simulink model "CLSfixed_pace"  (R2024b)
settings: Solver=FixedStepAuto  StartTime=0.0  StopTime=stoptime  FixedStep=stepsize  RelTol=1e-3
undefined symbols (not defined in the file or in its folder): AVI, cfg_length, LCP_delay, LRI, pNode_length, pPath_length, PVARP, stepsize, URI, VRP
libraries: Libs_unified x157
(part 2 of 3)

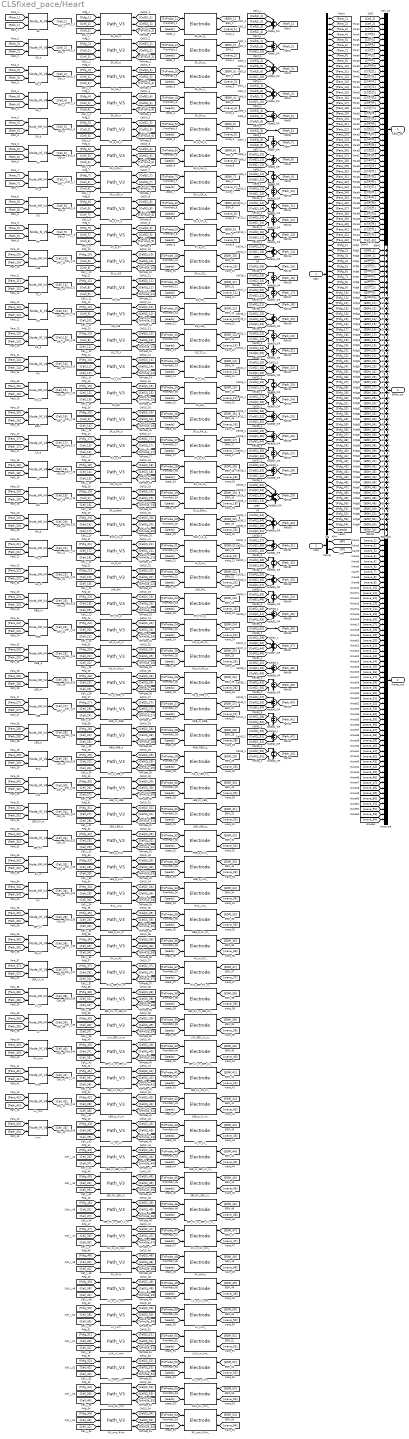
== system CLSfixed_pace/Heart ==
  Cfgin : Inport
  Pace : Inport  Port=2
  BH : Libs_unified/Node_NM_V4  SystemSampleTime=-1  VariantActivationTime=update diagram  AllowFlexibleInterface=on  Latency=0  AutoFrameSizeCalculation=off
  BH_His_p : Libs_unified/Path_V3  SystemSampleTime=-1  VariantActivationTime=update diagram  AllowFlexibleInterface=on  Latency=0  AutoFrameSizeCalculation=off
  BH_His_p_ : Libs_unified/Electrode  SystemSampleTime=-1  VariantActivationTime=update diagram  AllowFlexibleInterface=on  Latency=0  AutoFrameSizeCalculation=off
  Bach : Libs_unified/Node_M_V4  SystemSampleTime=-1  VariantActivationTime=update diagram  AllowFlexibleInterface=on  Latency=0  AutoFrameSizeCalculation=off
  Bach_LA_a : Libs_unified/Path_V3  SystemSampleTime=-1  VariantActivationTime=update diagram  AllowFlexibleInterface=on  Latency=0  AutoFrameSizeCalculation=off
  Bach_LA_a_ : Libs_unified/Electrode  SystemSampleTime=-1  VariantActivationTime=update diagram  AllowFlexibleInterface=on  Latency=0  AutoFrameSizeCalculation=off
  CN : Libs_unified/Node_N_V6  SystemSampleTime=-1  VariantActivationTime=update diagram  AllowFlexibleInterface=on  Latency=0  AutoFrameSizeCalculation=off
  CN_BH : Libs_unified/Path_V3  SystemSampleTime=-1  VariantActivationTime=update diagram  AllowFlexibleInterface=on  Latency=0  AutoFrameSizeCalculation=off
  CN_BH_ : Libs_unified/Electrode  SystemSampleTime=-1  VariantActivationTime=update diagram  AllowFlexibleInterface=on  Latency=0  AutoFrameSizeCalculation=off
  CS_LA : Libs_unified/Node_NM_V4  SystemSampleTime=-1  VariantActivationTime=update diagram  AllowFlexibleInterface=on  Latency=0  AutoFrameSizeCalculation=off
  CS_LV : Libs_unified/Node_M_V4  SystemSampleTime=-1  VariantActivationTime=update diagram  AllowFlexibleInterface=on  Latency=0  AutoFrameSizeCalculation=off
  CT : Libs_unified/Node_M_V4  SystemSampleTime=-1  VariantActivationTime=update diagram  AllowFlexibleInterface=on  Latency=0  AutoFrameSizeCalculation=off
  CT_a : Libs_unified/Node_NM_V4  SystemSampleTime=-1  VariantActivationTime=update diagram  AllowFlexibleInterface=on  Latency=0  AutoFrameSizeCalculation=off
  CT_a_CT : Libs_unified/Path_V3  SystemSampleTime=-1  VariantActivationTime=update diagram  AllowFlexibleInterface=on  Latency=0  AutoFrameSizeCalculation=off
  CT_a_CT_ : Libs_unified/Electrode  SystemSampleTime=-1  VariantActivationTime=update diagram  AllowFlexibleInterface=on  Latency=0  AutoFrameSizeCalculation=off
  Cell_out : Mux  Inputs=43
  Cfg : Demux  Outputs=[23,25,25,25,50,25,50,50,23,50,50,23,25,25,50,25,25,25,50,50,50,50,50,50,50,50,50,50,25,25,25,25,50,50,25,25,25,50,50,25,25,25,25,11,11,11,11,11,11,11,11,11,11,11,11,11,11,11,11,11,11,11,11,11,11,11,11,11,11,11,11,11,11,11,11,11,11,11,11,11,11,11,11,11,11,11,11,11,11,11,11,11,11,11,11,11,11,28]
  EGM_out : Sum  Inputs=54
  His_d : Libs_unified/Node_NM_V4  SystemSampleTime=-1  VariantActivationTime=update diagram  AllowFlexibleInterface=on  Latency=0  AutoFrameSizeCalculation=off
  His_d_LBB_m : Libs_unified/Path_V3  SystemSampleTime=-1  VariantActivationTime=update diagram  AllowFlexibleInterface=on  Latency=0  AutoFrameSizeCalculation=off
  His_d_LBB_m_ : Libs_unified/Electrode  SystemSampleTime=-1  VariantActivationTime=update diagram  AllowFlexibleInterface=on  Latency=0  AutoFrameSizeCalculation=off
  His_d_RBB_m : Libs_unified/Path_V3  SystemSampleTime=-1  VariantActivationTime=update diagram  AllowFlexibleInterface=on  Latency=0  AutoFrameSizeCalculation=off
  His_d_RBB_m_ : Libs_unified/Electrode  SystemSampleTime=-1  VariantActivationTime=update diagram  AllowFlexibleInterface=on  Latency=0  AutoFrameSizeCalculation=off
  His_m : Libs_unified/Node_NM_V4  SystemSampleTime=-1  VariantActivationTime=update diagram  AllowFlexibleInterface=on  Latency=0  AutoFrameSizeCalculation=off
  His_m_His_d : Libs_unified/Path_V3  SystemSampleTime=-1  VariantActivationTime=update diagram  AllowFlexibleInterface=on  Latency=0  AutoFrameSizeCalculation=off
  His_m_His_d_ : Libs_unified/Electrode  SystemSampleTime=-1  VariantActivationTime=update diagram  AllowFlexibleInterface=on  Latency=0  AutoFrameSizeCalculation=off
  His_p : Libs_unified/Node_NM_V4  SystemSampleTime=-1  VariantActivationTime=update diagram  AllowFlexibleInterface=on  Latency=0  AutoFrameSizeCalculation=off
  His_p_His_m : Libs_unified/Path_V3  SystemSampleTime=-1  VariantActivationTime=update diagram  AllowFlexibleInterface=on  Latency=0  AutoFrameSizeCalculation=off
  His_p_His_m_ : Libs_unified/Electrode  SystemSampleTime=-1  VariantActivationTime=update diagram  AllowFlexibleInterface=on  Latency=0  AutoFrameSizeCalculation=off
  LA : Libs_unified/Node_M_V4  SystemSampleTime=-1  VariantActivationTime=update diagram  AllowFlexibleInterface=on  Latency=0  AutoFrameSizeCalculation=off
  LA_a : Libs_unified/Node_M_V4  SystemSampleTime=-1  VariantActivationTime=update diagram  AllowFlexibleInterface=on  Latency=0  AutoFrameSizeCalculation=off
  LA_a_LA : Libs_unified/Path_V3  SystemSampleTime=-1  VariantActivationTime=update diagram  AllowFlexibleInterface=on  Latency=0  AutoFrameSizeCalculation=off
  LA_a_LA_ : Libs_unified/Electrode  SystemSampleTime=-1  VariantActivationTime=update diagram  AllowFlexibleInterface=on  Latency=0  AutoFrameSizeCalculation=off
  LBB : Libs_unified/Node_NM_V4  SystemSampleTime=-1  VariantActivationTime=update diagram  AllowFlexibleInterface=on  Latency=0  AutoFrameSizeCalculation=off
  LBB_LBB_a : Libs_unified/Path_V3  SystemSampleTime=-1  VariantActivationTime=update diagram  AllowFlexibleInterface=on  Latency=0  AutoFrameSizeCalculation=off
  LBB_LBB_a_ : Libs_unified/Electrode  SystemSampleTime=-1  VariantActivationTime=update diagram  AllowFlexibleInterface=on  Latency=0  AutoFrameSizeCalculation=off
  LBB_a : Libs_unified/Node_NM_V4  SystemSampleTime=-1  VariantActivationTime=update diagram  AllowFlexibleInterface=on  Latency=0  AutoFrameSizeCalculation=off
  LBB_a_LVA : Libs_unified/Path_V3  SystemSampleTime=-1  VariantActivationTime=update diagram  AllowFlexibleInterface=on  Latency=0  AutoFrameSizeCalculation=off
  LBB_a_LVA_ : Libs_unified/Electrode  SystemSampleTime=-1  VariantActivationTime=update diagram  AllowFlexibleInterface=on  Latency=0  AutoFrameSizeCalculation=off
  LBB_a_LV_m : Libs_unified/Path_V3  SystemSampleTime=-1  VariantActivationTime=update diagram  AllowFlexibleInterface=on  Latency=0  AutoFrameSizeCalculation=off
  LBB_a_LV_m_ : Libs_unified/Electrode  SystemSampleTime=-1  VariantActivationTime=update diagram  AllowFlexibleInterface=on  Latency=0  AutoFrameSizeCalculation=off
  LBB_m : Libs_unified/Node_NM_V4  SystemSampleTime=-1  VariantActivationTime=update diagram  AllowFlexibleInterface=on  Latency=0  AutoFrameSizeCalculation=off
  LBB_m_LBB : Libs_unified/Path_V3  SystemSampleTime=-1  VariantActivationTime=update diagram  AllowFlexibleInterface=on  Latency=0  AutoFrameSizeCalculation=off
  LBB_m_LBB_ : Libs_unified/Electrode  SystemSampleTime=-1  VariantActivationTime=update diagram  AllowFlexibleInterface=on  Latency=0  AutoFrameSizeCalculation=off
  LBB_m_SEP_LV_m : Libs_unified/Path_V3  SystemSampleTime=-1  VariantActivationTime=update diagram  AllowFlexibleInterface=on  Latency=0  AutoFrameSizeCalculation=off
  LBB_m_SEP_LV_m_ : Libs_unified/Electrode  SystemSampleTime=-1  VariantActivationTime=update diagram  AllowFlexibleInterface=on  Latency=0  AutoFrameSizeCalculation=off
  LNB : Libs_unified/Node_NM_V4  SystemSampleTime=-1  VariantActivationTime=update diagram  AllowFlexibleInterface=on  Latency=0  AutoFrameSizeCalculation=off
  LNB_BH : Libs_unified/Path_V3  SystemSampleTime=-1  VariantActivationTime=update diagram  AllowFlexibleInterface=on  Latency=0  AutoFrameSizeCalculation=off
  LNB_BH_ : Libs_unified/Electrode  SystemSampleTime=-1  VariantActivationTime=update diagram  AllowFlexibleInterface=on  Latency=0  AutoFrameSizeCalculation=off
  LV : Libs_unified/Node_NM_V4  SystemSampleTime=-1  VariantActivationTime=update diagram  AllowFlexibleInterface=on  Latency=0  AutoFrameSizeCalculation=off
  LVA : Libs_unified/Node_M_V4  SystemSampleTime=-1  VariantActivationTime=update diagram  AllowFlexibleInterface=on  Latency=0  AutoFrameSizeCalculation=off
  LVA_LV_mm : Libs_unified/Path_V3  SystemSampleTime=-1  VariantActivationTime=update diagram  AllowFlexibleInterface=on  Latency=0  AutoFrameSizeCalculation=off
  LVA_LV_mm_ : Libs_unified/Electrode  SystemSampleTime=-1  VariantActivationTime=update diagram  AllowFlexibleInterface=on  Latency=0  AutoFrameSizeCalculation=off
  LVA_SEP_LV_m : Libs_unified/Path_V3  SystemSampleTime=-1  VariantActivationTime=update diagram  AllowFlexibleInterface=on  Latency=0  AutoFrameSizeCalculation=off
  LVA_SEP_LV_m_ : Libs_unified/Electrode  SystemSampleTime=-1  VariantActivationTime=update diagram  AllowFlexibleInterface=on  Latency=0  AutoFrameSizeCalculation=off
  LV_LVm : Libs_unified/Path_V3  SystemSampleTime=-1  VariantActivationTime=update diagram  AllowFlexibleInterface=on  Latency=0  AutoFrameSizeCalculation=off
  LV_LVm_ : Libs_unified/Electrode  SystemSampleTime=-1  VariantActivationTime=update diagram  AllowFlexibleInterface=on  Latency=0  AutoFrameSizeCalculation=off
  LV_m : Libs_unified/Node_NM_V4  SystemSampleTime=-1  VariantActivationTime=update diagram  AllowFlexibleInterface=on  Latency=0  AutoFrameSizeCalculation=off
  LV_m_LV : Libs_unified/Path_V3  SystemSampleTime=-1  VariantActivationTime=update diagram  AllowFlexibleInterface=on  Latency=0  AutoFrameSizeCalculation=off
  LV_m_LV_ : Libs_unified/Electrode  SystemSampleTime=-1  VariantActivationTime=update diagram  AllowFlexibleInterface=on  Latency=0  AutoFrameSizeCalculation=off
  LV_m_LV_mm : Libs_unified/Path_V3  SystemSampleTime=-1  VariantActivationTime=update diagram  AllowFlexibleInterface=on  Latency=0  AutoFrameSizeCalculation=off
  LV_m_LV_mm_ : Libs_unified/Electrode  SystemSampleTime=-1  VariantActivationTime=update diagram  AllowFlexibleInterface=on  Latency=0  AutoFrameSizeCalculation=off
  LV_mm : Libs_unified/Node_M_V4  SystemSampleTime=-1  VariantActivationTime=update diagram  AllowFlexibleInterface=on  Latency=0  AutoFrameSizeCalculation=off
  LV_mm_LVm : Libs_unified/Path_V3  SystemSampleTime=-1  VariantActivationTime=update diagram  AllowFlexibleInterface=on  Latency=0  AutoFrameSizeCalculation=off
  LV_mm_LVm_ : Libs_unified/Electrode  SystemSampleTime=-1  VariantActivationTime=update diagram  AllowFlexibleInterface=on  Latency=0  AutoFrameSizeCalculation=off
  LVm : Libs_unified/Node_M_V4  SystemSampleTime=-1  VariantActivationTime=update diagram  AllowFlexibleInterface=on  Latency=0  AutoFrameSizeCalculation=off
  Node10_OR : Sum  Inputs=2
  Node11_OR : Sum  Inputs=2
  Node12_OR : Sum  Inputs=2
  Node13_OR : Sum  Inputs=2
  Node14_OR : Sum  Inputs=3
  Node16_OR : Sum  Inputs=2
  Node17_OR : Sum  Inputs=2
  Node19_OR : Sum  Inputs=3
  Node1_OR : Sum  Inputs=4
  Node20_OR : Sum  Inputs=2
  Node21_OR : Sum  Inputs=2
  Node22_OR : Sum  Inputs=3
  Node23_OR : Sum  Inputs=2
  Node24_OR : Sum  Inputs=2
  Node25_OR : Sum  Inputs=3
  Node26_OR : Sum  Inputs=3
  Node27_OR : Sum  Inputs=2
  Node28_OR : Sum  Inputs=3
  Node29_OR : Sum  Inputs=5
  Node2_OR : Sum  Inputs=3
  Node30_OR : Sum  Inputs=4
  Node31_OR : Sum  Inputs=3
  Node32_OR : Sum  Inputs=2
  Node33_OR : Sum  Inputs=3
  Node34_OR : Sum  Inputs=2
  Node35_OR : Sum  Inputs=3
  Node37_OR : Sum  Inputs=4
  Node38_OR : Sum  Inputs=3
  Node39_OR : Sum  Inputs=2
  Node3_OR : Sum  Inputs=4
  Node40_OR : Sum  Inputs=3
  Node41_OR : Sum  Inputs=2
  Node42_OR : Sum  Inputs=3
  Node43_OR : Sum  Inputs=2
  Node4_OR : Sum  Inputs=4
  Node5_OR : Sum  Inputs=3
  Node7_OR : Sum  Inputs=2
  Node8_OR : Sum  Inputs=3
  Node9_OR : Sum  Inputs=2
  OS : Libs_unified/Node_NM_V4  SystemSampleTime=-1  VariantActivationTime=update diagram  AllowFlexibleInterface=on  Latency=0  AutoFrameSizeCalculation=off
  OS_RE : Libs_unified/Path_V3  SystemSampleTime=-1  VariantActivationTime=update diagram  AllowFlexibleInterface=on  Latency=0  AutoFrameSizeCalculation=off
  OS_RE_ : Libs_unified/Electrode  SystemSampleTime=-1  VariantActivationTime=update diagram  AllowFlexibleInterface=on  Latency=0  AutoFrameSizeCalculation=off
  OS_TC_f : Libs_unified/Path_V3  SystemSampleTime=-1  VariantActivationTime=update diagram  AllowFlexibleInterface=on  Latency=0  AutoFrameSizeCalculation=off
  OS_TC_f_ : Libs_unified/Electrode  SystemSampleTime=-1  VariantActivationTime=update diagram  AllowFlexibleInterface=on  Latency=0  AutoFrameSizeCalculation=off
  Pacing : Demux  Outputs=2
  RA : Libs_unified/Node_M_V4  SystemSampleTime=-1  VariantActivationTime=update diagram  AllowFlexibleInterface=on  Latency=0  AutoFrameSizeCalculation=off
  RA_CS_LA : Libs_unified/Path_V3  SystemSampleTime=-1  VariantActivationTime=update diagram  AllowFlexibleInterface=on  Latency=0  AutoFrameSizeCalculation=off
  RA_CS_LA_ : Libs_unified/Electrode  SystemSampleTime=-1  VariantActivationTime=update diagram  AllowFlexibleInterface=on  Latency=0  AutoFrameSizeCalculation=off
  RA_a : Libs_unified/Node_M_V4  SystemSampleTime=-1  VariantActivationTime=update diagram  AllowFlexibleInterface=on  Latency=0  AutoFrameSizeCalculation=off
  RA_a_RA : Libs_unified/Path_V3  SystemSampleTime=-1  VariantActivationTime=update diagram  AllowFlexibleInterface=on  Latency=0  AutoFrameSizeCalculation=off
  RA_a_RA_ : Libs_unified/Electrode  SystemSampleTime=-1  VariantActivationTime=update diagram  AllowFlexibleInterface=on  Latency=0  AutoFrameSizeCalculation=off
  RBB : Libs_unified/Node_NM_V4  SystemSampleTime=-1  VariantActivationTime=update diagram  AllowFlexibleInterface=on  Latency=0  AutoFrameSizeCalculation=off
  RBB_RBB_a : Libs_unified/Path_V3  SystemSampleTime=-1  VariantActivationTime=update diagram  AllowFlexibleInterface=on  Latency=0  AutoFrameSizeCalculation=off
  RBB_RBB_a_ : Libs_unified/Electrode  SystemSampleTime=-1  VariantActivationTime=update diagram  AllowFlexibleInterface=on  Latency=0  AutoFrameSizeCalculation=off
  RBB_a : Libs_unified/Node_NM_V4  SystemSampleTime=-1  VariantActivationTime=update diagram  AllowFlexibleInterface=on  Latency=0  AutoFrameSizeCalculation=off
  RBB_a_RVA : Libs_unified/Path_V3  SystemSampleTime=-1  VariantActivationTime=update diagram  AllowFlexibleInterface=on  Latency=0  AutoFrameSizeCalculation=off
  RBB_a_RVA_ : Libs_unified/Electrode  SystemSampleTime=-1  VariantActivationTime=update diagram  AllowFlexibleInterface=on  Latency=0  AutoFrameSizeCalculation=off
  RBB_a_RV_m : Libs_unified/Path_V3  SystemSampleTime=-1  VariantActivationTime=update diagram  AllowFlexibleInterface=on  Latency=0  AutoFrameSizeCalculation=off
  RBB_a_RV_m_ : Libs_unified/Electrode  SystemSampleTime=-1  VariantActivationTime=update diagram  AllowFlexibleInterface=on  Latency=0  AutoFrameSizeCalculation=off
  RBB_m : Libs_unified/Node_NM_V4  SystemSampleTime=-1  VariantActivationTime=update diagram  AllowFlexibleInterface=on  Latency=0  AutoFrameSizeCalculation=off
  RBB_m_RBB : Libs_unified/Path_V3  SystemSampleTime=-1  VariantActivationTime=update diagram  AllowFlexibleInterface=on  Latency=0  AutoFrameSizeCalculation=off
  RBB_m_RBB_ : Libs_unified/Electrode  SystemSampleTime=-1  VariantActivationTime=update diagram  AllowFlexibleInterface=on  Latency=0  AutoFrameSizeCalculation=off
  RE : Libs_unified/Node_N_V6  SystemSampleTime=-1  VariantActivationTime=update diagram  AllowFlexibleInterface=on  Latency=0  AutoFrameSizeCalculation=off
  RE_LNB : Libs_unified/Path_V3  SystemSampleTime=-1  VariantActivationTime=update diagram  AllowFlexibleInterface=on  Latency=0  AutoFrameSizeCalculation=off
  RE_LNB_ : Libs_unified/Electrode  SystemSampleTime=-1  VariantActivationTime=update diagram  AllowFlexibleInterface=on  Latency=0  AutoFrameSizeCalculation=off
  RV : Libs_unified/Node_NM_V4  SystemSampleTime=-1  VariantActivationTime=update diagram  AllowFlexibleInterface=on  Latency=0  AutoFrameSizeCalculation=off
  RVA : Libs_unified/Node_M_V4  SystemSampleTime=-1  VariantActivationTime=update diagram  AllowFlexibleInterface=on  Latency=0  AutoFrameSizeCalculation=off
  RVA_LVA : Libs_unified/Path_V3  SystemSampleTime=-1  VariantActivationTime=update diagram  AllowFlexibleInterface=on  Latency=0  AutoFrameSizeCalculation=off
  RVA_LVA_ : Libs_unified/Electrode  SystemSampleTime=-1  VariantActivationTime=update diagram  AllowFlexibleInterface=on  Latency=0  AutoFrameSizeCalculation=off
  RVA_RV_mm : Libs_unified/Path_V3  SystemSampleTime=-1  VariantActivationTime=update diagram  AllowFlexibleInterface=on  Latency=0  AutoFrameSizeCalculation=off
  RVA_RV_mm_ : Libs_unified/Electrode  SystemSampleTime=-1  VariantActivationTime=update diagram  AllowFlexibleInterface=on  Latency=0  AutoFrameSizeCalculation=off
  RVA_SEP_RV_m : Libs_unified/Path_V3  SystemSampleTime=-1  VariantActivationTime=update diagram  AllowFlexibleInterface=on  Latency=0  AutoFrameSizeCalculation=off
  RVA_SEP_RV_m_ : Libs_unified/Electrode  SystemSampleTime=-1  VariantActivationTime=update diagram  AllowFlexibleInterface=on  Latency=0  AutoFrameSizeCalculation=off
  RV_RVm : Libs_unified/Path_V3  SystemSampleTime=-1  VariantActivationTime=update diagram  AllowFlexibleInterface=on  Latency=0  AutoFrameSizeCalculation=off
  RV_RVm_ : Libs_unified/Electrode  SystemSampleTime=-1  VariantActivationTime=update diagram  AllowFlexibleInterface=on  Latency=0  AutoFrameSizeCalculation=off
  RV_m : Libs_unified/Node_NM_V4  SystemSampleTime=-1  VariantActivationTime=update diagram  AllowFlexibleInterface=on  Latency=0  AutoFrameSizeCalculation=off
  RV_m_RV : Libs_unified/Path_V3  SystemSampleTime=-1  VariantActivationTime=update diagram  AllowFlexibleInterface=on  Latency=0  AutoFrameSizeCalculation=off
  RV_m_RV_ : Libs_unified/Electrode  SystemSampleTime=-1  VariantActivationTime=update diagram  AllowFlexibleInterface=on  Latency=0  AutoFrameSizeCalculation=off
  RV_m_RV_mm : Libs_unified/Path_V3  SystemSampleTime=-1  VariantActivationTime=update diagram  AllowFlexibleInterface=on  Latency=0  AutoFrameSizeCalculation=off
  RV_m_RV_mm_ : Libs_unified/Electrode  SystemSampleTime=-1  VariantActivationTime=update diagram  AllowFlexibleInterface=on  Latency=0  AutoFrameSizeCalculation=off
  RV_mm : Libs_unified/Node_M_V4  SystemSampleTime=-1  VariantActivationTime=update diagram  AllowFlexibleInterface=on  Latency=0  AutoFrameSizeCalculation=off
  RV_mm_RVm : Libs_unified/Path_V3  SystemSampleTime=-1  VariantActivationTime=update diagram  AllowFlexibleInterface=on  Latency=0  AutoFrameSizeCalculation=off
  RV_mm_RVm_ : Libs_unified/Electrode  SystemSampleTime=-1  VariantActivationTime=update diagram  AllowFlexibleInterface=on  Latency=0  AutoFrameSizeCalculation=off
  RVm : Libs_unified/Node_M_V4  SystemSampleTime=-1  VariantActivationTime=update diagram  AllowFlexibleInterface=on  Latency=0  AutoFrameSizeCalculation=off
  SA : Libs_unified/Node_N_V6  SystemSampleTime=-1  VariantActivationTime=update diagram  AllowFlexibleInterface=on  Latency=0  AutoFrameSizeCalculation=off
  SA_SA_a : Libs_unified/Path_V3  SystemSampleTime=-1  VariantActivationTime=update diagram  AllowFlexibleInterface=on  Latency=0  AutoFrameSizeCalculation=off
  SA_SA_a_ : Libs_unified/Electrode  SystemSampleTime=-1  VariantActivationTime=update diagram  AllowFlexibleInterface=on  Latency=0  AutoFrameSizeCalculation=off
  SA_SA_b : Libs_unified/Path_V3  SystemSampleTime=-1  VariantActivationTime=update diagram  AllowFlexibleInterface=on  Latency=0  AutoFrameSizeCalculation=off
  SA_SA_b_ : Libs_unified/Electrode  SystemSampleTime=-1  VariantActivationTime=update diagram  AllowFlexibleInterface=on  Latency=0  AutoFrameSizeCalculation=off
  SA_SA_c : Libs_unified/Path_V3  SystemSampleTime=-1  VariantActivationTime=update diagram  AllowFlexibleInterface=on  Latency=0  AutoFrameSizeCalculation=off
  SA_SA_c_ : Libs_unified/Electrode  SystemSampleTime=-1  VariantActivationTime=update diagram  AllowFlexibleInterface=on  Latency=0  AutoFrameSizeCalculation=off
  SA_SA_d : Libs_unified/Path_V3  SystemSampleTime=-1  VariantActivationTime=update diagram  AllowFlexibleInterface=on  Latency=0  AutoFrameSizeCalculation=off
  SA_SA_d_ : Libs_unified/Electrode  SystemSampleTime=-1  VariantActivationTime=update diagram  AllowFlexibleInterface=on  Latency=0  AutoFrameSizeCalculation=off
  SA_a : Libs_unified/Node_M_V4  SystemSampleTime=-1  VariantActivationTime=update diagram  AllowFlexibleInterface=on  Latency=0  AutoFrameSizeCalculation=off
  SA_a_Bach : Libs_unified/Path_V3  SystemSampleTime=-1  VariantActivationTime=update diagram  AllowFlexibleInterface=on  Latency=0  AutoFrameSizeCalculation=off
  SA_a_Bach_ : Libs_unified/Electrode  SystemSampleTime=-1  VariantActivationTime=update diagram  AllowFlexibleInterface=on  Latency=0  AutoFrameSizeCalculation=off
  SA_a_SA_b : Libs_unified/Path_V3  SystemSampleTime=-1  VariantActivationTime=update diagram  AllowFlexibleInterface=on  Latency=0  AutoFrameSizeCalculation=off
  SA_a_SA_b_ : Libs_unified/Electrode  SystemSampleTime=-1  VariantActivationTime=update diagram  AllowFlexibleInterface=on  Latency=0  AutoFrameSizeCalculation=off
  SA_b : Libs_unified/Node_M_V4  SystemSampleTime=-1  VariantActivationTime=update diagram  AllowFlexibleInterface=on  Latency=0  AutoFrameSizeCalculation=off
  SA_b_RA_a : Libs_unified/Path_V3  SystemSampleTime=-1  VariantActivationTime=update diagram  AllowFlexibleInterface=on  Latency=0  AutoFrameSizeCalculation=off
  SA_b_RA_a_ : Libs_unified/Electrode  SystemSampleTime=-1  VariantActivationTime=update diagram  AllowFlexibleInterface=on  Latency=0  AutoFrameSizeCalculation=off
  SA_b_SA_c : Libs_unified/Path_V3  SystemSampleTime=-1  VariantActivationTime=update diagram  AllowFlexibleInterface=on  Latency=0  AutoFrameSizeCalculation=off
  SA_b_SA_c_ : Libs_unified/Electrode  SystemSampleTime=-1  VariantActivationTime=update diagram  AllowFlexibleInterface=on  Latency=0  AutoFrameSizeCalculation=off
  SA_c : Libs_unified/Node_M_V4  SystemSampleTime=-1  VariantActivationTime=update diagram  AllowFlexibleInterface=on  Latency=0  AutoFrameSizeCalculation=off
  SA_c_OS : Libs_unified/Path_V3  SystemSampleTime=-1  VariantActivationTime=update diagram  AllowFlexibleInterface=on  Latency=0  AutoFrameSizeCalculation=off
  SA_c_OS_ : Libs_unified/Electrode  SystemSampleTime=-1  VariantActivationTime=update diagram  AllowFlexibleInterface=on  Latency=0  AutoFrameSizeCalculation=off
  SA_c_SA_d : Libs_unified/Path_V3  SystemSampleTime=-1  VariantActivationTime=update diagram  AllowFlexibleInterface=on  Latency=0  AutoFrameSizeCalculation=off
  SA_c_SA_d_ : Libs_unified/Electrode  SystemSampleTime=-1  VariantActivationTime=update diagram  AllowFlexibleInterface=on  Latency=0  AutoFrameSizeCalculation=off
  SA_d : Libs_unified/Node_NM_V4  SystemSampleTime=-1  VariantActivationTime=update diagram  AllowFlexibleInterface=on  Latency=0  AutoFrameSizeCalculation=off
  SA_d_CT_a : Libs_unified/Path_V3  SystemSampleTime=-1  VariantActivationTime=update diagram  AllowFlexibleInterface=on  Latency=0  AutoFrameSizeCalculation=off
  SA_d_CT_a_ : Libs_unified/Electrode  SystemSampleTime=-1  VariantActivationTime=update diagram  AllowFlexibleInterface=on  Latency=0  AutoFrameSizeCalculation=off
  SEP_LV : Libs_unified/Node_M_V4  SystemSampleTime=-1  VariantActivationTime=update diagram  AllowFlexibleInterface=on  Latency=0  AutoFrameSizeCalculation=off
  SEP_LV_CS_LV : Libs_unified/Path_V3  SystemSampleTime=-1  VariantActivationTime=update diagram  AllowFlexibleInterface=on  Latency=0  AutoFrameSizeCalculation=off
  SEP_LV_CS_LV_ : Libs_unified/Electrode  SystemSampleTime=-1  VariantActivationTime=update diagram  AllowFlexibleInterface=on  Latency=0  AutoFrameSizeCalculation=off
  SEP_LV_m : Libs_unified/Node_M_V4  SystemSampleTime=-1  VariantActivationTime=update diagram  AllowFlexibleInterface=on  Latency=0  AutoFrameSizeCalculation=off
  SEP_LV_m_SEP_LV : Libs_unified/Path_V3  SystemSampleTime=-1  VariantActivationTime=update diagram  AllowFlexibleInterface=on  Latency=0  AutoFrameSizeCalculation=off
  SEP_LV_m_SEP_LV_ : Libs_unified/Electrode  SystemSampleTime=-1  VariantActivationTime=update diagram  AllowFlexibleInterface=on  Latency=0  AutoFrameSizeCalculation=off
  SEP_RV : Libs_unified/Node_M_V4  SystemSampleTime=-1  VariantActivationTime=update diagram  AllowFlexibleInterface=on  Latency=0  AutoFrameSizeCalculation=off
  SEP_RV_SEP_LV : Libs_unified/Path_V3  SystemSampleTime=-1  VariantActivationTime=update diagram  AllowFlexibleInterface=on  Latency=0  AutoFrameSizeCalculation=off
  SEP_RV_SEP_LV_ : Libs_unified/Electrode  SystemSampleTime=-1  VariantActivationTime=update diagram  AllowFlexibleInterface=on  Latency=0  AutoFrameSizeCalculation=off
  SEP_RV_m : Libs_unified/Node_M_V4  SystemSampleTime=-1  VariantActivationTime=update diagram  AllowFlexibleInterface=on  Latency=0  AutoFrameSizeCalculation=off
  SEP_RV_m_SEP_LV_m : Libs_unified/Path_V3  SystemSampleTime=-1  VariantActivationTime=update diagram  AllowFlexibleInterface=on  Latency=0  AutoFrameSizeCalculation=off
  SEP_RV_m_SEP_LV_m_ : Libs_unified/Electrode  SystemSampleTime=-1  VariantActivationTime=update diagram  AllowFlexibleInterface=on  Latency=0  AutoFrameSizeCalculation=off
  SEP_RV_m_SEP_RV : Libs_unified/Path_V3  SystemSampleTime=-1  VariantActivationTime=update diagram  AllowFlexibleInterface=on  Latency=0  AutoFrameSizeCalculation=off
  SEP_RV_m_SEP_RV_ : Libs_unified/Electrode  SystemSampleTime=-1  VariantActivationTime=update diagram  AllowFlexibleInterface=on  Latency=0  AutoFrameSizeCalculation=off
  TC_f : Libs_unified/Node_NM_V4  SystemSampleTime=-1  VariantActivationTime=update diagram  AllowFlexibleInterface=on  Latency=0  AutoFrameSizeCalculation=off
  TC_f_CN : Libs_unified/Path_V3  SystemSampleTime=-1  VariantActivationTime=update diagram  AllowFlexibleInterface=on  Latency=0  AutoFrameSizeCalculation=off
  TC_f_CN_ : Libs_unified/Electrode  SystemSampleTime=-1  VariantActivationTime=update diagram  AllowFlexibleInterface=on  Latency=0  AutoFrameSizeCalculation=off
  Wave_out : Mux  Inputs=54
  Cells_out : Outport
  Waves_out : Outport  Port=2
  EGMs_out : Outport  Port=3
  wires:
  [wave_54] -> Wave_out/54
  [wave_53] -> Wave_out/53
  [wave_52] -> Wave_out/52
  [wave_51] -> Wave_out/51
  [wave_50] -> Wave_out/50
  [wave_49] -> Wave_out/49
  [wave_48] -> Wave_out/48
  [wave_47] -> Wave_out/47
  [wave_46] -> Wave_out/46
  [wave_45] -> Wave_out/45
  [wave_44] -> Wave_out/44
  [wave_43] -> Wave_out/43
  [wave_42] -> Wave_out/42
  [wave_41] -> Wave_out/41
  [wave_40] -> Wave_out/40
  [wave_39] -> Wave_out/39
  [wave_38] -> Wave_out/38
  [wave_37] -> Wave_out/37
  [wave_36] -> Wave_out/36
  [wave_35] -> Wave_out/35
  [wave_34] -> Wave_out/34
  [wave_33] -> Wave_out/33
  [wave_32] -> Wave_out/32
  [wave_31] -> Wave_out/31
  [wave_30] -> Wave_out/30
  [wave_29] -> Wave_out/29
  [wave_28] -> Wave_out/28
  [wave_27] -> Wave_out/27
  [wave_26] -> Wave_out/26
  [wave_25] -> Wave_out/25
  [wave_24] -> Wave_out/24
  [wave_23] -> Wave_out/23
  [wave_22] -> Wave_out/22
  [wave_21] -> Wave_out/21
  [wave_20] -> Wave_out/20
  [wave_19] -> Wave_out/19
  [wave_18] -> Wave_out/18
  [wave_17] -> Wave_out/17
  [wave_16] -> Wave_out/16
  [wave_15] -> Wave_out/15
  [wave_14] -> Wave_out/14
  [wave_13] -> Wave_out/13
  [wave_12] -> Wave_out/12
  [wave_11] -> Wave_out/11
  [wave_10] -> Wave_out/10
  [wave_9] -> Wave_out/9
  [wave_8] -> Wave_out/8
  [wave_7] -> Wave_out/7
  [wave_6] -> Wave_out/6
  [wave_5] -> Wave_out/5
  [wave_4] -> Wave_out/4
  [wave_3] -> Wave_out/3
  [wave_2] -> Wave_out/2
  [wave_1] -> Wave_out/1
  [EGM_54] -> EGM_out/54
  [EGM_53] -> EGM_out/53
  [EGM_52] -> EGM_out/52
  [EGM_51] -> EGM_out/51
  [EGM_50] -> EGM_out/50
  [EGM_49] -> EGM_out/49
  [EGM_48] -> EGM_out/48
  [EGM_47] -> EGM_out/47
  [EGM_46] -> EGM_out/46
  [EGM_45] -> EGM_out/45
  [EGM_44] -> EGM_out/44
  [EGM_43] -> EGM_out/43
  [EGM_42] -> EGM_out/42
  [EGM_41] -> EGM_out/41
  [EGM_40] -> EGM_out/40
  [EGM_39] -> EGM_out/39
  [EGM_38] -> EGM_out/38
  [EGM_37] -> EGM_out/37
  [EGM_36] -> EGM_out/36
  [EGM_35] -> EGM_out/35
  [EGM_34] -> EGM_out/34
  [EGM_33] -> EGM_out/33
  [EGM_32] -> EGM_out/32
  [EGM_31] -> EGM_out/31
  [EGM_30] -> EGM_out/30
  [EGM_29] -> EGM_out/29
  [EGM_28] -> EGM_out/28
  [EGM_27] -> EGM_out/27
  [EGM_26] -> EGM_out/26
  [EGM_25] -> EGM_out/25
  [EGM_24] -> EGM_out/24
  [EGM_23] -> EGM_out/23
  [EGM_22] -> EGM_out/22
  [EGM_21] -> EGM_out/21
  [EGM_20] -> EGM_out/20
  [EGM_19] -> EGM_out/19
  [EGM_18] -> EGM_out/18
  [EGM_17] -> EGM_out/17
  [EGM_16] -> EGM_out/16
  [EGM_15] -> EGM_out/15
  [EGM_14] -> EGM_out/14
  [EGM_13] -> EGM_out/13
  [EGM_12] -> EGM_out/12
  [EGM_11] -> EGM_out/11
  [EGM_10] -> EGM_out/10
  [EGM_9] -> EGM_out/9
  [EGM_8] -> EGM_out/8
  [EGM_7] -> EGM_out/7
  [EGM_6] -> EGM_out/6
  [EGM_5] -> EGM_out/5
  [EGM_4] -> EGM_out/4
  [EGM_3] -> EGM_out/3
  [EGM_2] -> EGM_out/2
  [EGM_1] -> EGM_out/1
  [Cell_43] -> Cell_out/43
  [Cell_42] -> Cell_out/42
  [Cell_41] -> Cell_out/41
  [Cell_40] -> Cell_out/40
  [Cell_39] -> Cell_out/39
  [Cell_38] -> Cell_out/38
  [Cell_37] -> Cell_out/37
  [Cell_36] -> Cell_out/36
  [Cell_35] -> Cell_out/35
  [Cell_34] -> Cell_out/34
  [Cell_33] -> Cell_out/33
  [Cell_32] -> Cell_out/32
  [Cell_31] -> Cell_out/31
  [Cell_30] -> Cell_out/30
  [Cell_29] -> Cell_out/29
  [Cell_28] -> Cell_out/28
  [Cell_27] -> Cell_out/27
  [Cell_26] -> Cell_out/26
  [Cell_25] -> Cell_out/25
  [Cell_24] -> Cell_out/24
  [Cell_23] -> Cell_out/23
  [Cell_22] -> Cell_out/22
  [Cell_21] -> Cell_out/21
  [Cell_20] -> Cell_out/20
  [Cell_19] -> Cell_out/19
  [Cell_18] -> Cell_out/18
  [Cell_17] -> Cell_out/17
  [Cell_16] -> Cell_out/16
  [Cell_15] -> Cell_out/15
  [Cell_14] -> Cell_out/14
  [Cell_13] -> Cell_out/13
  [Cell_12] -> Cell_out/12
  [Cell_11] -> Cell_out/11
  [Cell_10] -> Cell_out/10
  [Cell_9] -> Cell_out/9
  [Cell_8] -> Cell_out/8
  [Cell_7] -> Cell_out/7
  [Cell_6] -> Cell_out/6
  [Cell_5] -> Cell_out/5
  [Cell_4] -> Cell_out/4
  [Cell_3] -> Cell_out/3
  [Cell_2] -> Cell_out/2
  [Cell_1] -> Cell_out/1
  Wave_out/1 -> Waves_out/1
  EGM_out/1 -> EGMs_out/1
  Cell_out/1 -> Cells_out/1
  Pacing/2 -> [VP]
  Pacing/1 -> [AP]
  Cfg/98 -> [Leads]
  Cfg/97 -> [Pcfg_54]
  Cfg/96 -> [Pcfg_53]
  Cfg/95 -> [Pcfg_52]
  Cfg/94 -> [Pcfg_51]
  Cfg/93 -> [Pcfg_50]
  Cfg/92 -> [Pcfg_49]
  Cfg/91 -> [Pcfg_48]
  Cfg/90 -> [Pcfg_47]
  Cfg/89 -> [Pcfg_46]
  Cfg/88 -> [Pcfg_45]
  Cfg/87 -> [Pcfg_44]
  Cfg/86 -> [Pcfg_43]
  Cfg/85 -> [Pcfg_42]
  Cfg/84 -> [Pcfg_41]
  Cfg/83 -> [Pcfg_40]
  Cfg/82 -> [Pcfg_39]
  Cfg/81 -> [Pcfg_38]
  Cfg/80 -> [Pcfg_37]
  Cfg/79 -> [Pcfg_36]
  Cfg/78 -> [Pcfg_35]
  Cfg/77 -> [Pcfg_34]
  Cfg/76 -> [Pcfg_33]
  Cfg/75 -> [Pcfg_32]
  Cfg/74 -> [Pcfg_31]
  Cfg/73 -> [Pcfg_30]
  Cfg/72 -> [Pcfg_29]
  Cfg/71 -> [Pcfg_28]
  Cfg/70 -> [Pcfg_27]
  Cfg/69 -> [Pcfg_26]
  Cfg/68 -> [Pcfg_25]
  Cfg/67 -> [Pcfg_24]
  Cfg/66 -> [Pcfg_23]
  Cfg/65 -> [Pcfg_22]
  Cfg/64 -> [Pcfg_21]
  Cfg/63 -> [Pcfg_20]
  Cfg/62 -> [Pcfg_19]
  Cfg/61 -> [Pcfg_18]
  Cfg/60 -> [Pcfg_17]
  Cfg/59 -> [Pcfg_16]
  Cfg/58 -> [Pcfg_15]
  Cfg/57 -> [Pcfg_14]
  Cfg/56 -> [Pcfg_13]
  Cfg/55 -> [Pcfg_12]
  Cfg/54 -> [Pcfg_11]
  Cfg/53 -> [Pcfg_10]
  Cfg/52 -> [Pcfg_9]
  Cfg/51 -> [Pcfg_8]
  Cfg/50 -> [Pcfg_7]
  Cfg/49 -> [Pcfg_6]
  Cfg/48 -> [Pcfg_5]
  Cfg/47 -> [Pcfg_4]
  Cfg/46 -> [Pcfg_3]
  Cfg/45 -> [Pcfg_2]
  Cfg/44 -> [Pcfg_1]
  Cfg/43 -> [Para_43]
  Cfg/42 -> [Para_42]
  Cfg/41 -> [Para_41]
  Cfg/40 -> [Para_40]
  Cfg/39 -> [Para_39]
  Cfg/38 -> [Para_38]
  Cfg/37 -> [Para_37]
  Cfg/36 -> [Para_36]
  Cfg/35 -> [Para_35]
  Cfg/34 -> [Para_34]
  Cfg/33 -> [Para_33]
  Cfg/32 -> [Para_32]
  Cfg/31 -> [Para_31]
  Cfg/30 -> [Para_30]
  Cfg/29 -> [Para_29]
  Cfg/28 -> [Para_28]
  Cfg/27 -> [Para_27]
  Cfg/26 -> [Para_26]
  Cfg/25 -> [Para_25]
  Cfg/24 -> [Para_24]
  Cfg/23 -> [Para_23]
  Cfg/22 -> [Para_22]
  Cfg/21 -> [Para_21]
  Cfg/20 -> [Para_20]
  Cfg/19 -> [Para_19]
  Cfg/18 -> [Para_18]
  Cfg/17 -> [Para_17]
  Cfg/16 -> [Para_16]
  Cfg/15 -> [Para_15]
  Cfg/14 -> [Para_14]
  Cfg/13 -> [Para_13]
  Cfg/12 -> [Para_12]
  Cfg/11 -> [Para_11]
  Cfg/10 -> [Para_10]
  Cfg/9 -> [Para_9]
  Cfg/8 -> [Para_8]
  Cfg/7 -> [Para_7]
  Cfg/6 -> [Para_6]
  Cfg/5 -> [Para_5]
  Cfg/4 -> [Para_4]
  Cfg/3 -> [Para_3]
  Cfg/2 -> [Para_2]
  Cfg/1 -> [Para_1]
  Pace/1 -> Pacing/1
  Cfgin/1 -> Cfg/1
  Node43_OR/1 -> [Path_43]
  [Celli2j_52] -> Node43_OR/2
  [Celli2j_50] -> Node43_OR/1
  Node42_OR/1 -> [Path_42]
  [Cellj2i_52] -> Node42_OR/3
  [Celli2j_51] -> Node42_OR/2
  [Celli2j_49] -> Node42_OR/1
  Node41_OR/1 -> [Path_41]
  [Celli2j_54] -> Node41_OR/2
  [Celli2j_48] -> Node41_OR/1
  Node40_OR/1 -> [Path_40]
  [Cellj2i_54] -> Node40_OR/3
  [Celli2j_53] -> Node40_OR/2
  [Celli2j_47] -> Node40_OR/1
  Node39_OR/1 -> [Path_39]
  [Cellj2i_50] -> Node39_OR/2
  [Celli2j_43] -> Node39_OR/1
  Node38_OR/1 -> [Path_38]
  [Cellj2i_49] -> Node38_OR/3
  [Cellj2i_43] -> Node38_OR/2
  [Celli2j_42] -> Node38_OR/1
  Node37_OR/1 -> [Path_37]
  [Celli2j_46] -> Node37_OR/4
  [Celli2j_44] -> Node37_OR/3
  [Cellj2i_40] -> Node37_OR/2
  [Celli2j_39] -> Node37_OR/1
  [Celli2j_41] -> [Path_36]
  Node35_OR/1 -> [Path_35]
  [Celli2j_45] -> Node35_OR/3
  [Cellj2i_41] -> Node35_OR/2
  [Celli2j_40] -> Node35_OR/1
  Node34_OR/1 -> [Path_34]
  [Cellj2i_48] -> Node34_OR/2
  [Celli2j_36] -> Node34_OR/1
  Node33_OR/1 -> [Path_33]
  [Cellj2i_47] -> Node33_OR/3
  [Cellj2i_36] -> Node33_OR/2
  [Celli2j_35] -> Node33_OR/1
  Node32_OR/1 -> [Path_32]
  [Cellj2i_45] -> Node32_OR/2
  [Celli2j_38] -> Node32_OR/1
  Node31_OR/1 -> [Path_31]
  [Cellj2i_46] -> Node31_OR/3
  [Cellj2i_38] -> Node31_OR/2
  [Celli2j_37] -> Node31_OR/1
  Node30_OR/1 -> [Path_30]
  [Cellj2i_51] -> Node30_OR/4
  [Cellj2i_39] -> Node30_OR/3
  [Celli2j_34] -> Node30_OR/2
  [Celli2j_33] -> Node30_OR/1
  [VP] -> Node29_OR/5
  Node29_OR/1 -> [Path_29]
  [Cellj2i_53] -> Node29_OR/4
  [Cellj2i_37] -> Node29_OR/3
  [Cellj2i_34] -> Node29_OR/2
  [Celli2j_32] -> Node29_OR/1
  Node28_OR/1 -> [Path_28]
  [Cellj2i_42] -> Node28_OR/3
  [Cellj2i_33] -> Node28_OR/2
  [Celli2j_31] -> Node28_OR/1
  Node27_OR/1 -> [Path_27]
  [Cellj2i_31] -> Node27_OR/2
  [Celli2j_30] -> Node27_OR/1
  Node26_OR/1 -> [Path_26]
  [Cellj2i_44] -> Node26_OR/3
  [Cellj2i_30] -> Node26_OR/2
  [Celli2j_29] -> Node26_OR/1
  Node25_OR/1 -> [Path_25]
  [Cellj2i_35] -> Node25_OR/3
  [Cellj2i_32] -> Node25_OR/2
  [Celli2j_28] -> Node25_OR/1
  Node24_OR/1 -> [Path_24]
  [Cellj2i_28] -> Node24_OR/2
  [Celli2j_27] -> Node24_OR/1
  Node23_OR/1 -> [Path_23]
  [Cellj2i_27] -> Node23_OR/2
  [Celli2j_26] -> Node23_OR/1
  Node22_OR/1 -> [Path_22]
  [Cellj2i_29] -> Node22_OR/3
  [Cellj2i_26] -> Node22_OR/2
  [Celli2j_25] -> Node22_OR/1
  Node21_OR/1 -> [Path_21]
  [Cellj2i_25] -> Node21_OR/2
  [Celli2j_24] -> Node21_OR/1
  Node20_OR/1 -> [Path_20]
  [Cellj2i_24] -> Node20_OR/2
  [Celli2j_23] -> Node20_OR/1
  Node19_OR/1 -> [Path_19]
  [Cellj2i_23] -> Node19_OR/3
  [Celli2j_22] -> Node19_OR/2
  [Celli2j_15] -> Node19_OR/1
  [Celli2j_21] -> [Path_18]
  Node17_OR/1 -> [Path_17]
  [Cellj2i_21] -> Node17_OR/2
  [Celli2j_20] -> Node17_OR/1
  Node16_OR/1 -> [Path_16]
  [Cellj2i_20] -> Node16_OR/2
  [Celli2j_19] -> Node16_OR/1
  [Celli2j_18] -> [Path_15]
  [AP] -> Node14_OR/3
  Node14_OR/1 -> [Path_14]
  [Cellj2i_18] -> Node14_OR/2
  [Celli2j_17] -> Node14_OR/1
  Node13_OR/1 -> [Path_13]
  [Cellj2i_17] -> Node13_OR/2
  [Celli2j_16] -> Node13_OR/1
  Node12_OR/1 -> [Path_12]
  [Cellj2i_15] -> Node12_OR/2
  [Celli2j_14] -> Node12_OR/1
  Node11_OR/1 -> [Path_11]
  [Cellj2i_14] -> Node11_OR/2
  [Celli2j_13] -> Node11_OR/1
  Node10_OR/1 -> [Path_10]
  [Cellj2i_22] -> Node10_OR/2
  [Celli2j_12] -> Node10_OR/1
  Node9_OR/1 -> [Path_9]
  [Cellj2i_12] -> Node9_OR/2
  [Celli2j_11] -> Node9_OR/1
  Node8_OR/1 -> [Path_8]
  [Cellj2i_13] -> Node8_OR/3
  [Cellj2i_11] -> Node8_OR/2
  [Celli2j_10] -> Node8_OR/1
  Node7_OR/1 -> [Path_7]
  [Cellj2i_9] -> Node7_OR/2
  [Celli2j_8] -> Node7_OR/1
  [Celli2j_9] -> [Path_6]
  Node5_OR/1 -> [Path_5]
  [Cellj2i_8] -> Node5_OR/3
  [Celli2j_7] -> Node5_OR/2
  [Celli2j_4] -> Node5_OR/1
  Node4_OR/1 -> [Path_4]
  [Cellj2i_10] -> Node4_OR/4
  [Cellj2i_7] -> Node4_OR/3
  [Celli2j_6] -> Node4_OR/2
  [Celli2j_3] -> Node4_OR/1
  Node3_OR/1 -> [Path_3]
  [Cellj2i_16] -> Node3_OR/4
  [Cellj2i_6] -> Node3_OR/3
  [Celli2j_5] -> Node3_OR/2
  [Celli2j_2] -> Node3_OR/1
  Node2_OR/1 -> [Path_2]
  [Cellj2i_19] -> Node2_OR/3
  [Cellj2i_5] -> Node2_OR/2
  [Celli2j_1] -> Node2_OR/1
  Node1_OR/1 -> [Path_1]
  [Cellj2i_4] -> Node1_OR/4
  [Cellj2i_3] -> Node1_OR/3
  [Cellj2i_2] -> Node1_OR/2
  [Cellj2i_1] -> Node1_OR/1
  [Leads] -> RV_mm_RVm_/2
  [ToProbe_54] -> RV_mm_RVm_/1
  RV_mm_RVm_/2 -> [wave_54]
  RV_mm_RVm_/1 -> [EGM_54]
  [Leads] -> RVA_RV_mm_/2
  [ToProbe_53] -> RVA_RV_mm_/1
  RVA_RV_mm_/2 -> [wave_53]
  RVA_RV_mm_/1 -> [EGM_53]
  [Leads] -> LV_mm_LVm_/2
  [ToProbe_52] -> LV_mm_LVm_/1
  LV_mm_LVm_/2 -> [wave_52]
  LV_mm_LVm_/1 -> [EGM_52]
  [Leads] -> LVA_LV_mm_/2
  [ToProbe_51] -> LVA_LV_mm_/1
  LVA_LV_mm_/2 -> [wave_51]
  LVA_LV_mm_/1 -> [EGM_51]
  [Leads] -> LV_LVm_/2
  [ToProbe_50] -> LV_LVm_/1
  LV_LVm_/2 -> [wave_50]
  LV_LVm_/1 -> [EGM_50]
  [Leads] -> LV_m_LV_mm_/2
  [ToProbe_49] -> LV_m_LV_mm_/1
  LV_m_LV_mm_/2 -> [wave_49]
  LV_m_LV_mm_/1 -> [EGM_49]
  [Leads] -> RV_RVm_/2
  [ToProbe_48] -> RV_RVm_/1
  RV_RVm_/2 -> [wave_48]
  RV_RVm_/1 -> [EGM_48]
  [Leads] -> RV_m_RV_mm_/2
  [ToProbe_47] -> RV_m_RV_mm_/1
  RV_m_RV_mm_/2 -> [wave_47]
  RV_m_RV_mm_/1 -> [EGM_47]
  [Leads] -> SEP_RV_m_SEP_LV_m_/2
  [ToProbe_46] -> SEP_RV_m_SEP_LV_m_/1
  SEP_RV_m_SEP_LV_m_/2 -> [wave_46]
  SEP_RV_m_SEP_LV_m_/1 -> [EGM_46]
  [Leads] -> SEP_RV_SEP_LV_/2
  [ToProbe_45] -> SEP_RV_SEP_LV_/1
  SEP_RV_SEP_LV_/2 -> [wave_45]
  SEP_RV_SEP_LV_/1 -> [EGM_45]
  [Leads] -> LBB_m_SEP_LV_m_/2
  [ToProbe_44] -> LBB_m_SEP_LV_m_/1
  LBB_m_SEP_LV_m_/2 -> [wave_44]
  LBB_m_SEP_LV_m_/1 -> [EGM_44]
  [Leads] -> LV_m_LV_/2
  [ToProbe_43] -> LV_m_LV_/1
  LV_m_LV_/2 -> [wave_43]
  LV_m_LV_/1 -> [EGM_43]
  [Leads] -> LBB_a_LV_m_/2
  [ToProbe_42] -> LBB_a_LV_m_/1
  LBB_a_LV_m_/2 -> [wave_42]
  LBB_a_LV_m_/1 -> [EGM_42]
  [Leads] -> SEP_LV_CS_LV_/2
  [ToProbe_41] -> SEP_LV_CS_LV_/1
  SEP_LV_CS_LV_/2 -> [wave_41]
  SEP_LV_CS_LV_/1 -> [EGM_41]
  [Leads] -> SEP_LV_m_SEP_LV_/2
  [ToProbe_40] -> SEP_LV_m_SEP_LV_/1
  SEP_LV_m_SEP_LV_/2 -> [wave_40]
  SEP_LV_m_SEP_LV_/1 -> [EGM_40]
  [Leads] -> LVA_SEP_LV_m_/2
  [ToProbe_39] -> LVA_SEP_LV_m_/1
  LVA_SEP_LV_m_/2 -> [wave_39]
  LVA_SEP_LV_m_/1 -> [EGM_39]
  [Leads] -> SEP_RV_m_SEP_RV_/2
  [ToProbe_38] -> SEP_RV_m_SEP_RV_/1
  SEP_RV_m_SEP_RV_/2 -> [wave_38]
  SEP_RV_m_SEP_RV_/1 -> [EGM_38]
  [Leads] -> RVA_SEP_RV_m_/2
  [ToProbe_37] -> RVA_SEP_RV_m_/1
  RVA_SEP_RV_m_/2 -> [wave_37]
  RVA_SEP_RV_m_/1 -> [EGM_37]
  [Leads] -> RV_m_RV_/2
  [ToProbe_36] -> RV_m_RV_/1
  RV_m_RV_/2 -> [wave_36]
  RV_m_RV_/1 -> [EGM_36]
  [Leads] -> RBB_a_RV_m_/2
  [ToProbe_35] -> RBB_a_RV_m_/1
  RBB_a_RV_m_/2 -> [wave_35]
  RBB_a_RV_m_/1 -> [EGM_35]
  [Leads] -> RVA_LVA_/2
  [ToProbe_34] -> RVA_LVA_/1
  RVA_LVA_/2 -> [wave_34]
  RVA_LVA_/1 -> [EGM_34]
  [Leads] -> LBB_a_LVA_/2
  [ToProbe_33] -> LBB_a_LVA_/1
  LBB_a_LVA_/2 -> [wave_33]
  LBB_a_LVA_/1 -> [EGM_33]
  [Leads] -> RBB_a_RVA_/2
  [ToProbe_32] -> RBB_a_RVA_/1
  RBB_a_RVA_/2 -> [wave_32]
  RBB_a_RVA_/1 -> [EGM_32]
  [Leads] -> LBB_LBB_a_/2
  [ToProbe_31] -> LBB_LBB_a_/1
  LBB_LBB_a_/2 -> [wave_31]
  LBB_LBB_a_/1 -> [EGM_31]
  [Leads] -> LBB_m_LBB_/2
  [ToProbe_30] -> LBB_m_LBB_/1
  LBB_m_LBB_/2 -> [wave_30]
  LBB_m_LBB_/1 -> [EGM_30]
  [Leads] -> His_d_LBB_m_/2
  [ToProbe_29] -> His_d_LBB_m_/1
  His_d_LBB_m_/2 -> [wave_29]
  His_d_LBB_m_/1 -> [EGM_29]
  [Leads] -> RBB_RBB_a_/2
  [ToProbe_28] -> RBB_RBB_a_/1
  RBB_RBB_a_/2 -> [wave_28]
  RBB_RBB_a_/1 -> [EGM_28]
  [Leads] -> RBB_m_RBB_/2
  [ToProbe_27] -> RBB_m_RBB_/1
  RBB_m_RBB_/2 -> [wave_27]
  RBB_m_RBB_/1 -> [EGM_27]
  [Leads] -> His_d_RBB_m_/2
  [ToProbe_26] -> His_d_RBB_m_/1
  His_d_RBB_m_/2 -> [wave_26]
  His_d_RBB_m_/1 -> [EGM_26]
  [Leads] -> His_m_His_d_/2
  [ToProbe_25] -> His_m_His_d_/1
  His_m_His_d_/2 -> [wave_25]
  His_m_His_d_/1 -> [EGM_25]
  [Leads] -> His_p_His_m_/2
  [ToProbe_24] -> His_p_His_m_/1
  His_p_His_m_/2 -> [wave_24]
  His_p_His_m_/1 -> [EGM_24]
  [Leads] -> BH_His_p_/2
  [ToProbe_23] -> BH_His_p_/1
  BH_His_p_/2 -> [wave_23]
  BH_His_p_/1 -> [EGM_23]
  [Leads] -> LNB_BH_/2
  [ToProbe_22] -> LNB_BH_/1
  LNB_BH_/2 -> [wave_22]
  LNB_BH_/1 -> [EGM_22]
  [Leads] -> LA_a_LA_/2
  [ToProbe_21] -> LA_a_LA_/1
  LA_a_LA_/2 -> [wave_21]
  LA_a_LA_/1 -> [EGM_21]
  [Leads] -> Bach_LA_a_/2
  [ToProbe_20] -> Bach_LA_a_/1
  Bach_LA_a_/2 -> [wave_20]
  Bach_LA_a_/1 -> [EGM_20]
  [Leads] -> SA_a_Bach_/2
  [ToProbe_19] -> SA_a_Bach_/1
  SA_a_Bach_/2 -> [wave_19]
  SA_a_Bach_/1 -> [EGM_19]
  [Leads] -> RA_CS_LA_/2
  [ToProbe_18] -> RA_CS_LA_/1
  RA_CS_LA_/2 -> [wave_18]
  RA_CS_LA_/1 -> [EGM_18]
  [Leads] -> RA_a_RA_/2
  [ToProbe_17] -> RA_a_RA_/1
  RA_a_RA_/2 -> [wave_17]
  RA_a_RA_/1 -> [EGM_17]
  [Leads] -> SA_b_RA_a_/2
  [ToProbe_16] -> SA_b_RA_a_/1
  SA_b_RA_a_/2 -> [wave_16]
  SA_b_RA_a_/1 -> [EGM_16]
  [Leads] -> CN_BH_/2
  [ToProbe_15] -> CN_BH_/1
  CN_BH_/2 -> [wave_15]
  CN_BH_/1 -> [EGM_15]
  [Leads] -> TC_f_CN_/2
  [ToProbe_14] -> TC_f_CN_/1
  TC_f_CN_/2 -> [wave_14]
  TC_f_CN_/1 -> [EGM_14]
  [Leads] -> OS_TC_f_/2
  [ToProbe_13] -> OS_TC_f_/1
  OS_TC_f_/2 -> [wave_13]
  OS_TC_f_/1 -> [EGM_13]
  [Leads] -> RE_LNB_/2
  [ToProbe_12] -> RE_LNB_/1
  RE_LNB_/2 -> [wave_12]
  RE_LNB_/1 -> [EGM_12]
  [Leads] -> OS_RE_/2
  [ToProbe_11] -> OS_RE_/1
  OS_RE_/2 -> [wave_11]
  OS_RE_/1 -> [EGM_11]
  [Leads] -> SA_c_OS_/2
  [ToProbe_10] -> SA_c_OS_/1
  SA_c_OS_/2 -> [wave_10]
  SA_c_OS_/1 -> [EGM_10]
  [Leads] -> CT_a_CT_/2
  [ToProbe_9] -> CT_a_CT_/1
  CT_a_CT_/2 -> [wave_9]
  CT_a_CT_/1 -> [EGM_9]
  [Leads] -> SA_d_CT_a_/2
  [ToProbe_8] -> SA_d_CT_a_/1
  SA_d_CT_a_/2 -> [wave_8]
  SA_d_CT_a_/1 -> [EGM_8]
  [Leads] -> SA_c_SA_d_/2
  [ToProbe_7] -> SA_c_SA_d_/1
  SA_c_SA_d_/2 -> [wave_7]
  SA_c_SA_d_/1 -> [EGM_7]
  [Leads] -> SA_b_SA_c_/2
  [ToProbe_6] -> SA_b_SA_c_/1
  SA_b_SA_c_/2 -> [wave_6]
  SA_b_SA_c_/1 -> [EGM_6]
  [Leads] -> SA_a_SA_b_/2
  [ToProbe_5] -> SA_a_SA_b_/1
  SA_a_SA_b_/2 -> [wave_5]
  SA_a_SA_b_/1 -> [EGM_5]
  [Leads] -> SA_SA_d_/2
  [ToProbe_4] -> SA_SA_d_/1
  SA_SA_d_/2 -> [wave_4]
  SA_SA_d_/1 -> [EGM_4]
  [Leads] -> SA_SA_c_/2
  [ToProbe_3] -> SA_SA_c_/1
  SA_SA_c_/2 -> [wave_3]
  SA_SA_c_/1 -> [EGM_3]
  [Leads] -> SA_SA_b_/2
  [ToProbe_2] -> SA_SA_b_/1
  SA_SA_b_/2 -> [wave_2]
  SA_SA_b_/1 -> [EGM_2]
  [Leads] -> SA_SA_a_/2
  [ToProbe_1] -> SA_SA_a_/1
  SA_SA_a_/2 -> [wave_1]
  SA_SA_a_/1 -> [EGM_1]
  [Cell_41] -> RV_mm_RVm/3
  [Cell_40] -> RV_mm_RVm/2
  [Pcfg_54] -> RV_mm_RVm/1
  RV_mm_RVm/3 -> [ToProbe_54]
  RV_mm_RVm/2 -> [Celli2j_54]
  RV_mm_RVm/1 -> [Cellj2i_54]
  [Cell_40] -> RVA_RV_mm/3
  [Cell_29] -> RVA_RV_mm/2
  [Pcfg_53] -> RVA_RV_mm/1
  RVA_RV_mm/3 -> [ToProbe_53]
  RVA_RV_mm/2 -> [Celli2j_53]
  RVA_RV_mm/1 -> [Cellj2i_53]
  [Cell_43] -> LV_mm_LVm/3
  [Cell_42] -> LV_mm_LVm/2
  [Pcfg_52] -> LV_mm_LVm/1
  LV_mm_LVm/3 -> [ToProbe_52]
  LV_mm_LVm/2 -> [Celli2j_52]
  LV_mm_LVm/1 -> [Cellj2i_52]
  [Cell_42] -> LVA_LV_mm/3
  [Cell_30] -> LVA_LV_mm/2
  [Pcfg_51] -> LVA_LV_mm/1
  LVA_LV_mm/3 -> [ToProbe_51]
  LVA_LV_mm/2 -> [Celli2j_51]
  LVA_LV_mm/1 -> [Cellj2i_51]
  [Cell_43] -> LV_LVm/3
  [Cell_39] -> LV_LVm/2
  [Pcfg_50] -> LV_LVm/1
  LV_LVm/3 -> [ToProbe_50]
  LV_LVm/2 -> [Celli2j_50]
  LV_LVm/1 -> [Cellj2i_50]
  [Cell_42] -> LV_m_LV_mm/3
  [Cell_38] -> LV_m_LV_mm/2
  [Pcfg_49] -> LV_m_LV_mm/1
  LV_m_LV_mm/3 -> [ToProbe_49]
  LV_m_LV_mm/2 -> [Celli2j_49]
  LV_m_LV_mm/1 -> [Cellj2i_49]
  [Cell_41] -> RV_RVm/3
  [Cell_34] -> RV_RVm/2
  [Pcfg_48] -> RV_RVm/1
  RV_RVm/3 -> [ToProbe_48]
  RV_RVm/2 -> [Celli2j_48]
  RV_RVm/1 -> [Cellj2i_48]
  [Cell_40] -> RV_m_RV_mm/3
  [Cell_33] -> RV_m_RV_mm/2
  [Pcfg_47] -> RV_m_RV_mm/1
  RV_m_RV_mm/3 -> [ToProbe_47]
  RV_m_RV_mm/2 -> [Celli2j_47]
  RV_m_RV_mm/1 -> [Cellj2i_47]
  [Cell_37] -> SEP_RV_m_SEP_LV_m/3
  [Cell_31] -> SEP_RV_m_SEP_LV_m/2
  [Pcfg_46] -> SEP_RV_m_SEP_LV_m/1
  SEP_RV_m_SEP_LV_m/3 -> [ToProbe_46]
  SEP_RV_m_SEP_LV_m/2 -> [Celli2j_46]
  SEP_RV_m_SEP_LV_m/1 -> [Cellj2i_46]
  [Cell_35] -> SEP_RV_SEP_LV/3
  [Cell_32] -> SEP_RV_SEP_LV/2
  [Pcfg_45] -> SEP_RV_SEP_LV/1
  SEP_RV_SEP_LV/3 -> [ToProbe_45]
  SEP_RV_SEP_LV/2 -> [Celli2j_45]
  SEP_RV_SEP_LV/1 -> [Cellj2i_45]
  [Cell_37] -> LBB_m_SEP_LV_m/3
  [Cell_26] -> LBB_m_SEP_LV_m/2
  [Pcfg_44] -> LBB_m_SEP_LV_m/1
  LBB_m_SEP_LV_m/3 -> [ToProbe_44]
  LBB_m_SEP_LV_m/2 -> [Celli2j_44]
  LBB_m_SEP_LV_m/1 -> [Cellj2i_44]
  [Cell_39] -> LV_m_LV/3
  [Cell_38] -> LV_m_LV/2
  [Pcfg_43] -> LV_m_LV/1
  LV_m_LV/3 -> [ToProbe_43]
  LV_m_LV/2 -> [Celli2j_43]
  LV_m_LV/1 -> [Cellj2i_43]
  [Cell_38] -> LBB_a_LV_m/3
  [Cell_28] -> LBB_a_LV_m/2
  [Pcfg_42] -> LBB_a_LV_m/1
  LBB_a_LV_m/3 -> [ToProbe_42]
  LBB_a_LV_m/2 -> [Celli2j_42]
  LBB_a_LV_m/1 -> [Cellj2i_42]
  [Cell_36] -> SEP_LV_CS_LV/3
  [Cell_35] -> SEP_LV_CS_LV/2
  [Pcfg_41] -> SEP_LV_CS_LV/1
  SEP_LV_CS_LV/3 -> [ToProbe_41]
  SEP_LV_CS_LV/2 -> [Celli2j_41]
  SEP_LV_CS_LV/1 -> [Cellj2i_41]
  [Cell_35] -> SEP_LV_m_SEP_LV/3
  [Cell_37] -> SEP_LV_m_SEP_LV/2
  [Pcfg_40] -> SEP_LV_m_SEP_LV/1
  SEP_LV_m_SEP_LV/3 -> [ToProbe_40]
  SEP_LV_m_SEP_LV/2 -> [Celli2j_40]
  SEP_LV_m_SEP_LV/1 -> [Cellj2i_40]
  [Cell_37] -> LVA_SEP_LV_m/3
  [Cell_30] -> LVA_SEP_LV_m/2
  [Pcfg_39] -> LVA_SEP_LV_m/1
  LVA_SEP_LV_m/3 -> [ToProbe_39]
  LVA_SEP_LV_m/2 -> [Celli2j_39]
  LVA_SEP_LV_m/1 -> [Cellj2i_39]
  [Cell_32] -> SEP_RV_m_SEP_RV/3
  [Cell_31] -> SEP_RV_m_SEP_RV/2
  [Pcfg_38] -> SEP_RV_m_SEP_RV/1
  SEP_RV_m_SEP_RV/3 -> [ToProbe_38]
  SEP_RV_m_SEP_RV/2 -> [Celli2j_38]
  SEP_RV_m_SEP_RV/1 -> [Cellj2i_38]
  [Cell_31] -> RVA_SEP_RV_m/3
  [Cell_29] -> RVA_SEP_RV_m/2
  [Pcfg_37] -> RVA_SEP_RV_m/1
  RVA_SEP_RV_m/3 -> [ToProbe_37]
  RVA_SEP_RV_m/2 -> [Celli2j_37]
  RVA_SEP_RV_m/1 -> [Cellj2i_37]
  [Cell_34] -> RV_m_RV/3
  [Cell_33] -> RV_m_RV/2
  [Pcfg_36] -> RV_m_RV/1
  RV_m_RV/3 -> [ToProbe_36]
  RV_m_RV/2 -> [Celli2j_36]
  RV_m_RV/1 -> [Cellj2i_36]
  [Cell_33] -> RBB_a_RV_m/3
  [Cell_25] -> RBB_a_RV_m/2
  [Pcfg_35] -> RBB_a_RV_m/1
  RBB_a_RV_m/3 -> [ToProbe_35]
  RBB_a_RV_m/2 -> [Celli2j_35]
  RBB_a_RV_m/1 -> [Cellj2i_35]
  [Cell_30] -> RVA_LVA/3
  [Cell_29] -> RVA_LVA/2
  [Pcfg_34] -> RVA_LVA/1
  RVA_LVA/3 -> [ToProbe_34]
  RVA_LVA/2 -> [Celli2j_34]
  RVA_LVA/1 -> [Cellj2i_34]
  [Cell_30] -> LBB_a_LVA/3
  [Cell_28] -> LBB_a_LVA/2
  [Pcfg_33] -> LBB_a_LVA/1
  LBB_a_LVA/3 -> [ToProbe_33]
  LBB_a_LVA/2 -> [Celli2j_33]
  LBB_a_LVA/1 -> [Cellj2i_33]
  [Cell_29] -> RBB_a_RVA/3
  [Cell_25] -> RBB_a_RVA/2
  [Pcfg_32] -> RBB_a_RVA/1
  RBB_a_RVA/3 -> [ToProbe_32]
  RBB_a_RVA/2 -> [Celli2j_32]
  RBB_a_RVA/1 -> [Cellj2i_32]
  [Cell_28] -> LBB_LBB_a/3
  [Cell_27] -> LBB_LBB_a/2
  [Pcfg_31] -> LBB_LBB_a/1
  LBB_LBB_a/3 -> [ToProbe_31]
  LBB_LBB_a/2 -> [Celli2j_31]
  LBB_LBB_a/1 -> [Cellj2i_31]
  [Cell_27] -> LBB_m_LBB/3
  [Cell_26] -> LBB_m_LBB/2
  [Pcfg_30] -> LBB_m_LBB/1
  LBB_m_LBB/3 -> [ToProbe_30]
  LBB_m_LBB/2 -> [Celli2j_30]
  LBB_m_LBB/1 -> [Cellj2i_30]
  [Cell_26] -> His_d_LBB_m/3
  [Cell_22] -> His_d_LBB_m/2
  [Pcfg_29] -> His_d_LBB_m/1
  His_d_LBB_m/3 -> [ToProbe_29]
  His_d_LBB_m/2 -> [Celli2j_29]
  His_d_LBB_m/1 -> [Cellj2i_29]
  [Cell_25] -> RBB_RBB_a/3
  [Cell_24] -> RBB_RBB_a/2
  [Pcfg_28] -> RBB_RBB_a/1
  RBB_RBB_a/3 -> [ToProbe_28]
  RBB_RBB_a/2 -> [Celli2j_28]
  RBB_RBB_a/1 -> [Cellj2i_28]
  [Cell_24] -> RBB_m_RBB/3
  [Cell_23] -> RBB_m_RBB/2
  [Pcfg_27] -> RBB_m_RBB/1
  RBB_m_RBB/3 -> [ToProbe_27]
  RBB_m_RBB/2 -> [Celli2j_27]
  RBB_m_RBB/1 -> [Cellj2i_27]
  [Cell_23] -> His_d_RBB_m/3
  [Cell_22] -> His_d_RBB_m/2
  [Pcfg_26] -> His_d_RBB_m/1
  His_d_RBB_m/3 -> [ToProbe_26]
  His_d_RBB_m/2 -> [Celli2j_26]
  His_d_RBB_m/1 -> [Cellj2i_26]
  [Cell_22] -> His_m_His_d/3
  [Cell_21] -> His_m_His_d/2
  [Pcfg_25] -> His_m_His_d/1
  His_m_His_d/3 -> [ToProbe_25]
  His_m_His_d/2 -> [Celli2j_25]
  His_m_His_d/1 -> [Cellj2i_25]
  [Cell_21] -> His_p_His_m/3
  [Cell_20] -> His_p_His_m/2
  [Pcfg_24] -> His_p_His_m/1
  His_p_His_m/3 -> [ToProbe_24]
  His_p_His_m/2 -> [Celli2j_24]
  His_p_His_m/1 -> [Cellj2i_24]
  [Cell_20] -> BH_His_p/3
  [Cell_19] -> BH_His_p/2
  [Pcfg_23] -> BH_His_p/1
  BH_His_p/3 -> [ToProbe_23]
  BH_His_p/2 -> [Celli2j_23]
  BH_His_p/1 -> [Cellj2i_23]
  [Cell_19] -> LNB_BH/3
  [Cell_10] -> LNB_BH/2
  [Pcfg_22] -> LNB_BH/1
  LNB_BH/3 -> [ToProbe_22]
  LNB_BH/2 -> [Celli2j_22]
  LNB_BH/1 -> [Cellj2i_22]
  [Cell_18] -> LA_a_LA/3
  [Cell_17] -> LA_a_LA/2
  [Pcfg_21] -> LA_a_LA/1
  LA_a_LA/3 -> [ToProbe_21]
  LA_a_LA/2 -> [Celli2j_21]
  LA_a_LA/1 -> [Cellj2i_21]
  [Cell_17] -> Bach_LA_a/3
  [Cell_16] -> Bach_LA_a/2
  [Pcfg_20] -> Bach_LA_a/1
  Bach_LA_a/3 -> [ToProbe_20]
  Bach_LA_a/2 -> [Celli2j_20]
  Bach_LA_a/1 -> [Cellj2i_20]
  [Cell_16] -> SA_a_Bach/3
  [Cell_2] -> SA_a_Bach/2
  [Pcfg_19] -> SA_a_Bach/1
  SA_a_Bach/3 -> [ToProbe_19]
  SA_a_Bach/2 -> [Celli2j_19]
  SA_a_Bach/1 -> [Cellj2i_19]
  [Cell_15] -> RA_CS_LA/3
  [Cell_14] -> RA_CS_LA/2
  [Pcfg_18] -> RA_CS_LA/1
  RA_CS_LA/3 -> [ToProbe_18]
  RA_CS_LA/2 -> [Celli2j_18]
  RA_CS_LA/1 -> [Cellj2i_18]
  [Cell_14] -> RA_a_RA/3
  [Cell_13] -> RA_a_RA/2
  [Pcfg_17] -> RA_a_RA/1
  RA_a_RA/3 -> [ToProbe_17]
  RA_a_RA/2 -> [Celli2j_17]
  RA_a_RA/1 -> [Cellj2i_17]
  [Cell_13] -> SA_b_RA_a/3
  [Cell_3] -> SA_b_RA_a/2
  [Pcfg_16] -> SA_b_RA_a/1
  SA_b_RA_a/3 -> [ToProbe_16]
  SA_b_RA_a/2 -> [Celli2j_16]
  SA_b_RA_a/1 -> [Cellj2i_16]
  [Cell_19] -> CN_BH/3
  [Cell_12] -> CN_BH/2
  [Pcfg_15] -> CN_BH/1
  CN_BH/3 -> [ToProbe_15]
  CN_BH/2 -> [Celli2j_15]
  CN_BH/1 -> [Cellj2i_15]
  [Cell_12] -> TC_f_CN/3
  [Cell_11] -> TC_f_CN/2
  [Pcfg_14] -> TC_f_CN/1
  TC_f_CN/3 -> [ToProbe_14]
  TC_f_CN/2 -> [Celli2j_14]
  TC_f_CN/1 -> [Cellj2i_14]
  [Cell_11] -> OS_TC_f/3
  [Cell_8] -> OS_TC_f/2
  [Pcfg_13] -> OS_TC_f/1
  OS_TC_f/3 -> [ToProbe_13]
  OS_TC_f/2 -> [Celli2j_13]
  OS_TC_f/1 -> [Cellj2i_13]
  [Cell_10] -> RE_LNB/3
  [Cell_9] -> RE_LNB/2
  [Pcfg_12] -> RE_LNB/1
  RE_LNB/3 -> [ToProbe_12]
  RE_LNB/2 -> [Celli2j_12]
  RE_LNB/1 -> [Cellj2i_12]
  [Cell_9] -> OS_RE/3
  [Cell_8] -> OS_RE/2
  [Pcfg_11] -> OS_RE/1
  OS_RE/3 -> [ToProbe_11]
  OS_RE/2 -> [Celli2j_11]
  OS_RE/1 -> [Cellj2i_11]
  [Cell_8] -> SA_c_OS/3
  [Cell_4] -> SA_c_OS/2
  [Pcfg_10] -> SA_c_OS/1
  SA_c_OS/3 -> [ToProbe_10]
  SA_c_OS/2 -> [Celli2j_10]
  SA_c_OS/1 -> [Cellj2i_10]
  [Cell_6] -> CT_a_CT/3
  [Cell_7] -> CT_a_CT/2
  [Pcfg_9] -> CT_a_CT/1
  CT_a_CT/3 -> [ToProbe_9]
  CT_a_CT/2 -> [Celli2j_9]
  CT_a_CT/1 -> [Cellj2i_9]
  [Cell_7] -> SA_d_CT_a/3
  [Cell_5] -> SA_d_CT_a/2
  [Pcfg_8] -> SA_d_CT_a/1
  SA_d_CT_a/3 -> [ToProbe_8]
  SA_d_CT_a/2 -> [Celli2j_8]
  SA_d_CT_a/1 -> [Cellj2i_8]
  [Cell_5] -> SA_c_SA_d/3
  [Cell_4] -> SA_c_SA_d/2
  [Pcfg_7] -> SA_c_SA_d/1
  SA_c_SA_d/3 -> [ToProbe_7]
  SA_c_SA_d/2 -> [Celli2j_7]
  SA_c_SA_d/1 -> [Cellj2i_7]
  [Cell_4] -> SA_b_SA_c/3
  [Cell_3] -> SA_b_SA_c/2
  [Pcfg_6] -> SA_b_SA_c/1
  SA_b_SA_c/3 -> [ToProbe_6]
  SA_b_SA_c/2 -> [Celli2j_6]
  SA_b_SA_c/1 -> [Cellj2i_6]
  [Cell_3] -> SA_a_SA_b/3
  [Cell_2] -> SA_a_SA_b/2
  [Pcfg_5] -> SA_a_SA_b/1
  SA_a_SA_b/3 -> [ToProbe_5]
  SA_a_SA_b/2 -> [Celli2j_5]
  SA_a_SA_b/1 -> [Cellj2i_5]
  [Cell_5] -> SA_SA_d/3
  [Cell_1] -> SA_SA_d/2
  [Pcfg_4] -> SA_SA_d/1
  SA_SA_d/3 -> [ToProbe_4]
  SA_SA_d/2 -> [Celli2j_4]
  SA_SA_d/1 -> [Cellj2i_4]
  [Cell_4] -> SA_SA_c/3
  [Cell_1] -> SA_SA_c/2
  [Pcfg_3] -> SA_SA_c/1
  SA_SA_c/3 -> [ToProbe_3]
  SA_SA_c/2 -> [Celli2j_3]
  SA_SA_c/1 -> [Cellj2i_3]
  [Cell_3] -> SA_SA_b/3
  [Cell_1] -> SA_SA_b/2
  [Pcfg_2] -> SA_SA_b/1
  SA_SA_b/3 -> [ToProbe_2]
  SA_SA_b/2 -> [Celli2j_2]
  SA_SA_b/1 -> [Cellj2i_2]
  [Cell_2] -> SA_SA_a/3
  [Cell_1] -> SA_SA_a/2
  [Pcfg_1] -> SA_SA_a/1
  SA_SA_a/3 -> [ToProbe_1]
  SA_SA_a/2 -> [Celli2j_1]
  SA_SA_a/1 -> [Cellj2i_1]
  [Path_43] -> LVm/2
  [Para_43] -> LVm/1
  LVm/1 -> [Cell_43]
  [Path_42] -> LV_mm/2
  [Para_42] -> LV_mm/1
  LV_mm/1 -> [Cell_42]
  [Path_41] -> RVm/2
  [Para_41] -> RVm/1
  RVm/1 -> [Cell_41]
  [Path_40] -> RV_mm/2
  [Para_40] -> RV_mm/1
  RV_mm/1 -> [Cell_40]
  [Path_39] -> LV/2
  [Para_39] -> LV/1
  LV/1 -> [Cell_39]
  [Path_38] -> LV_m/2
  [Para_38] -> LV_m/1
  LV_m/1 -> [Cell_38]
  [Path_37] -> SEP_LV_m/2
  [Para_37] -> SEP_LV_m/1
  SEP_LV_m/1 -> [Cell_37]
  [Path_36] -> CS_LV/2
  [Para_36] -> CS_LV/1
  CS_LV/1 -> [Cell_36]
  [Path_35] -> SEP_LV/2
  [Para_35] -> SEP_LV/1
  SEP_LV/1 -> [Cell_35]
  [Path_34] -> RV/2
  [Para_34] -> RV/1
  RV/1 -> [Cell_34]
  [Path_33] -> RV_m/2
  [Para_33] -> RV_m/1
  RV_m/1 -> [Cell_33]
  [Path_32] -> SEP_RV/2
  [Para_32] -> SEP_RV/1
  SEP_RV/1 -> [Cell_32]
  [Path_31] -> SEP_RV_m/2
  [Para_31] -> SEP_RV_m/1
  SEP_RV_m/1 -> [Cell_31]
  [Path_30] -> LVA/2
  [Para_30] -> LVA/1
  LVA/1 -> [Cell_30]
  [Path_29] -> RVA/2
  [Para_29] -> RVA/1
  RVA/1 -> [Cell_29]
  [Path_28] -> LBB_a/2
  [Para_28] -> LBB_a/1
  LBB_a/1 -> [Cell_28]
  [Path_27] -> LBB/2
  [Para_27] -> LBB/1
  LBB/1 -> [Cell_27]
  [Path_26] -> LBB_m/2
  [Para_26] -> LBB_m/1
  LBB_m/1 -> [Cell_26]
  [Path_25] -> RBB_a/2
  [Para_25] -> RBB_a/1
  RBB_a/1 -> [Cell_25]
  [Path_24] -> RBB/2
  [Para_24] -> RBB/1
  RBB/1 -> [Cell_24]
  [Path_23] -> RBB_m/2
  [Para_23] -> RBB_m/1
  RBB_m/1 -> [Cell_23]
  [Path_22] -> His_d/2
  [Para_22] -> His_d/1
  His_d/1 -> [Cell_22]
  [Path_21] -> His_m/2
  [Para_21] -> His_m/1
  His_m/1 -> [Cell_21]
  [Path_20] -> His_p/2
  [Para_20] -> His_p/1
  His_p/1 -> [Cell_20]
  [Path_19] -> BH/2
  [Para_19] -> BH/1
  BH/1 -> [Cell_19]
  [Path_18] -> LA/2
  [Para_18] -> LA/1
  LA/1 -> [Cell_18]
  [Path_17] -> LA_a/2
  [Para_17] -> LA_a/1
  LA_a/1 -> [Cell_17]
  [Path_16] -> Bach/2
  [Para_16] -> Bach/1
  Bach/1 -> [Cell_16]
  [Path_15] -> CS_LA/2
  [Para_15] -> CS_LA/1
  CS_LA/1 -> [Cell_15]
  [Path_14] -> RA/2
  [Para_14] -> RA/1
  RA/1 -> [Cell_14]
  [Path_13] -> RA_a/2
  [Para_13] -> RA_a/1
  RA_a/1 -> [Cell_13]
  [Path_12] -> CN/2
  [Para_12] -> CN/1
  CN/1 -> [Cell_12]
  [Path_11] -> TC_f/2
  [Para_11] -> TC_f/1
  TC_f/1 -> [Cell_11]
  [Path_10] -> LNB/2
  [Para_10] -> LNB/1
  LNB/1 -> [Cell_10]
  [Path_9] -> RE/2
  [Para_9] -> RE/1
  RE/1 -> [Cell_9]
  [Path_8] -> OS/2
  [Para_8] -> OS/1
  OS/1 -> [Cell_8]
  [Path_7] -> CT_a/2
  [Para_7] -> CT_a/1
  CT_a/1 -> [Cell_7]
  [Path_6] -> CT/2
  [Para_6] -> CT/1
  CT/1 -> [Cell_6]
  [Path_5] -> SA_d/2
  [Para_5] -> SA_d/1
  SA_d/1 -> [Cell_5]
  [Path_4] -> SA_c/2
  [Para_4] -> SA_c/1
  SA_c/1 -> [Cell_4]
  [Path_3] -> SA_b/2
  [Para_3] -> SA_b/1
  SA_b/1 -> [Cell_3]
  [Path_2] -> SA_a/2
  [Para_2] -> SA_a/1
  SA_a/1 -> [Cell_2]
  [Path_1] -> SA/2
  [Para_1] -> SA/1
  SA/1 -> [Cell_1]
